simulink model "Simulink_DobleP"  (R2022a)
settings: Solver=VariableStepAuto  StartTime=0.0  StopTime=10.0  MaxStep=0.01  RelTol=1e-3
values from neighbouring files (symbols this model uses):
  g = 9.81    [Constantes_DobleP.m]
  l1 = 0.3    [Constantes_DobleP.m]
  l2 = 0.25    [Constantes_DobleP.m]
  m1 = 0.2    [Constantes_DobleP.m]
  m2 = 0.1    [Constantes_DobleP.m]
settings Model: Creator=jamez  LastModifiedBy=jamez

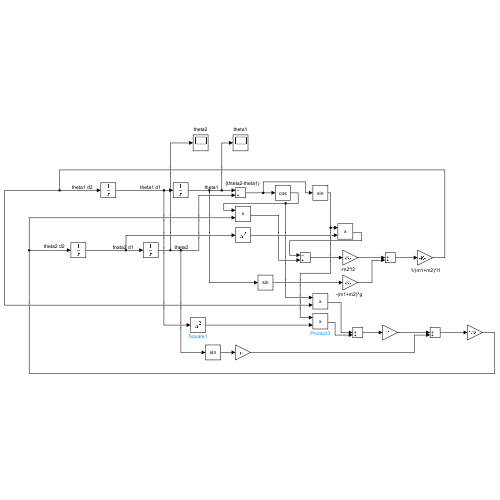
[thumbnail: Simulink's stored preview of the top-level diagram]
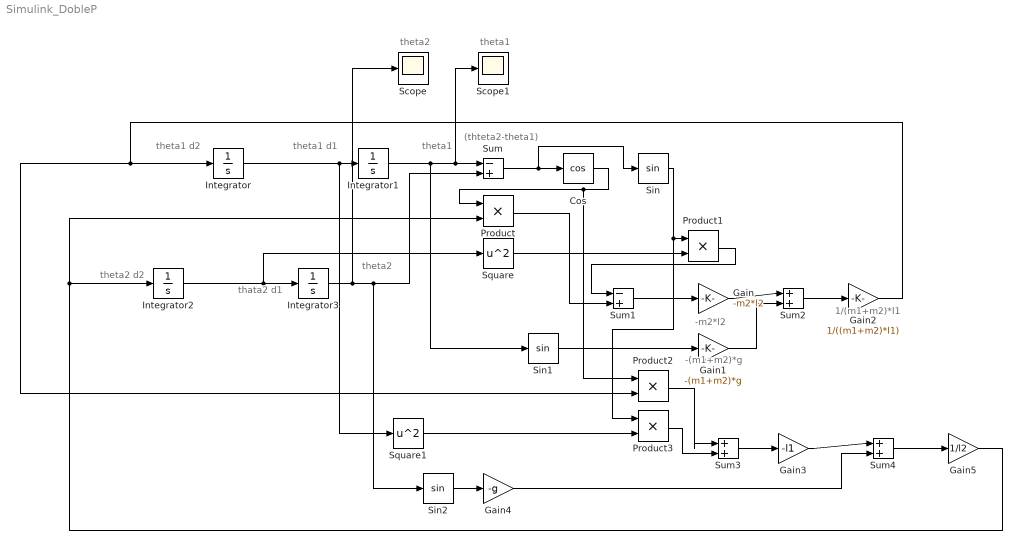
== system Simulink_DobleP ==
  note: theta1
  note: theta2
  note: theta2 d2
  note: theta1 d2
  note: 1/(m1+m2)*l1
  note: -m2*l2
  note: (thteta2-theta1)
  note: theta1
  note: theta1 d1
  note: thata2 d1
  note: theta2
  note: -(m1+m2)*g
  Cos : Trigonometry  Operator=cos
  Gain : Gain  Gain=-m2*l2
  Gain1 : Gain  Gain=-(m1+m2)*g
  Gain2 : Gain  Gain=1/((m1+m2)*l1)
  Gain3 : Gain  Gain=-l1
  Gain4 : Gain  Gain=-g
  Gain5 : Gain  Gain=1/l2
  Integrator : Integrator
  Integrator1 : Integrator
  Integrator2 : Integrator
  Integrator3 : Integrator  InitialCondition=(35*pi)/180
  Product{,1..3} (4 alike) : Product
  Scope : Scope
  Scope1 : Scope
  Sin : Trigonometry
  Sin1 : Trigonometry
  Sin2 : Trigonometry
  Square : Math  Operator=square
  Square1 : Math  Operator=square
  Sum : Sum  Inputs=-+
  Sum1 : Sum  Inputs=-+
  Sum2 : Sum  Inputs=|++
  Sum3 : Sum  Inputs=|++
  Sum4 : Sum  Inputs=|++
  wires:
  Integrator/1 -> Square1/1, Integrator1/1
  Integrator1/1 -> Sin1/1, Scope1/1, Sum/1
  Integrator2/1 -> Square/1, Integrator3/1
  Integrator3/1 -> Sum/2, Sin2/1, Scope/1
  Sum/1 -> Sin/1, Cos/1
  Gain5/1 -> Integrator2/1, Product/2
  Cos/1 -> Product2/1, Product/1
  Square/1 -> Product1/2
  Sin/1 -> Product3/1, Product1/1
  Product1/1 -> Sum1/1
  Product/1 -> Sum1/2
  Sum1/1 -> Gain/1
  Gain/1 -> Sum2/1
  Sin1/1 -> Gain1/1
  Gain1/1 -> Sum2/2
  Sum2/1 -> Gain2/1
  Gain2/1 -> Product2/2, Integrator/1
  Square1/1 -> Product3/2
  Product3/1 -> Sum3/2
  Product2/1 -> Sum3/1
  Sum3/1 -> Gain3/1
  Gain3/1 -> Sum4/1
  Gain4/1 -> Sum4/2
  Sum4/1 -> Gain5/1
  Sin2/1 -> Gain4/1
